simulink model "flash_adc"  (R2022a)
settings: Solver=VariableStepAuto  StartTime=0.0  StopTime=10  FixedStep=0.01  RelTol=1e-3
libraries: dspxfrm3 x1, msbAdcArchitectures x1, msbAdcFoundation x1
settings Model: Creator=jonathan  LastModifiedBy=jonathan

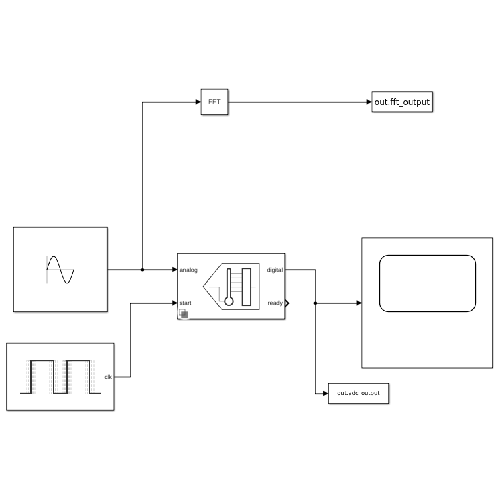
[thumbnail: Simulink's stored preview of the top-level diagram]
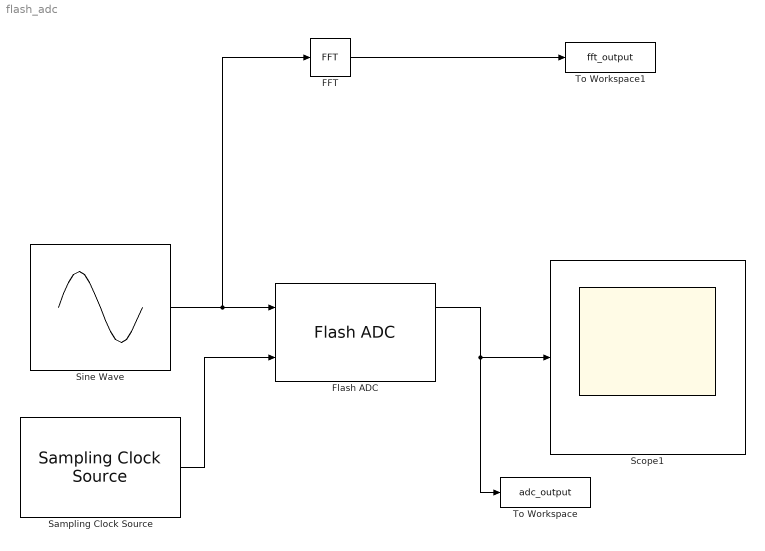
== system flash_adc ==
  FFT : dspxfrm3/FFT  FFTImplementation=Auto  CompMethod=Table lookup  TableOpt=NEW  TableOptActive=Speed  BitRevOrder=off  Normalize=off  InheritFFTLength=off  FFTLength=1024  WrapInput=on  roundingMode=Floor  overflowMode=off  firstCoeffDataTypeStr=Inherit: Same word length as input  firstCoeffLastDataTypeStr=Inherit: Same word length as input  outputMin=[]  outputMax=[]
  Flash ADC : msbAdcArchitectures/Flash ADC  LabelModeActiveChoice=Simulink Blocks  NBits=8  InputRange=[-1 1]  ExtStartClk=on  StartFreq=1e6  StartClkJitter=1e-12  SampleInterval=0.25e-6  Trigger=Rising edge  MatchScale=on  OutputPolarity=Auto  OutDataType=double  SimulateUsing=Simulink blocks  EnableImp=off  OffsetError=0  OffsetErrorUnit=LSB  GainError=0  GainErrorUnit=LSB  Bubbles=[]
      settings: SourceProductBaseCode=AM
  Sampling Clock Source : msbAdcFoundation/Sampling Clock Source  Freq=1e4  Min=0  Max=1  RmsJitt=1e-12  CustomSeed=off  Seed=0  CustomInitialOutput=off  InitialOutput=1  ExtraBuffer=off  NBuffer=50
      settings: SourceProductBaseCode=AM  SignalType=Square wave
  Scope1 : Scope
  Sine Wave : Sin  SampleTime=0
  To Workspace : ToWorkspace  VariableName=adc_output  SampleTime=-1
  To Workspace1 : ToWorkspace  VariableName=fft_output  SampleTime=-1
  wires:
  Flash ADC/1 -> To Workspace/1, Scope1/1
  Sine Wave/1 -> FFT/1, Flash ADC/1
  Sampling Clock Source/1 -> Flash ADC/2
  FFT/1 -> To Workspace1/1
